simulink model "DiscreteDiffSwerveModuleSimulation"  (R2022a)
settings: Solver=VariableStepAuto  StartTime=0.0  StopTime=2.0  RelTol=1e-3
values from neighbouring files (symbols this model uses):
  Kff = pinv(sysd.B)    [DiffSwerveChassis.m]    (also in GetDiffSwerveModule.m; RunDiffSwerveSimulation.m)
  lqr_K = lqr(sysd, Q, R)    [DiffSwerveChassis.m]    (also in GetDiffSwerveModule.m; RunDiffSwerveSimulation.m)
  sysd = c2d(sysc, Ts)    [DiffSwerveChassis.m]    (also in GetDiffSwerveModule.m; RunDiffSwerveSimulation.m)
  Ts = 0.005    [DiffSwerveChassis.m]    (also in GetDiffSwerveModule.m; RunDiffSwerveSimulation.m)
settings Model: Creator=benjaminwarwick  LastModifiedBy=woz4t

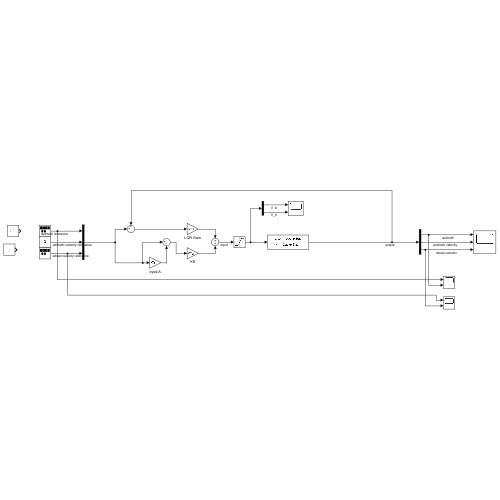
[thumbnail: Simulink's stored preview of the top-level diagram]
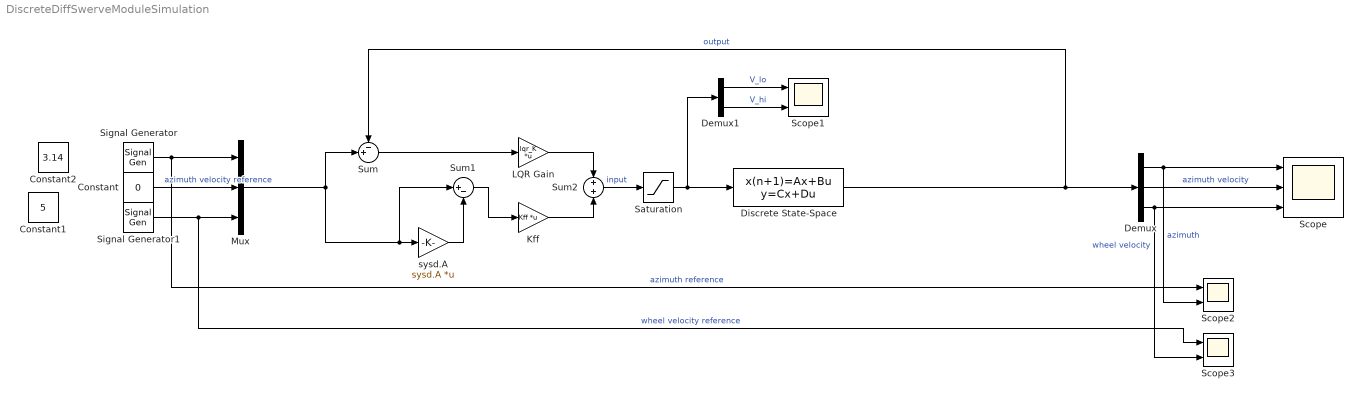
== system DiscreteDiffSwerveModuleSimulation ==
  Constant : Constant  Value=0
  Constant1 : Constant  Value=5
  Constant2 : Constant  Value=3.14
  Demux : Demux  Outputs=3
  Demux1 : Demux  Outputs=2
  Discrete State-Space : DiscreteStateSpace  A=sysd.A  B=sysd.B  C=sysd.C  D=sysd.D  SampleTime=Ts
  Kff : Gain  Gain=Kff  Multiplication=Matrix(K*u)
  LQR Gain : Gain  Gain=lqr_K  Multiplication=Matrix(K*u)
  Mux : Mux  Inputs=3
  Saturation : Saturate  UpperLimit=12  LowerLimit=-12
  Scope : Scope  NumInputPorts=3
  Scope1 : Scope  NumInputPorts=2
  Scope2 : Scope  NumInputPorts=2
  Scope3 : Scope  NumInputPorts=2
  Signal Generator : SignalGenerator  WaveForm=square  Amplitude=3.14  Frequency=20  Units=rad/sec
  Signal Generator1 : SignalGenerator  WaveForm=square  Amplitude=5  Frequency=20  Units=rad/sec
  Sum : Sum  Inputs=-+|
  Sum1 : Sum  Inputs=|+-
  Sum2 : Sum
  sysd.A : Gain  Gain=sysd.A  Multiplication=Matrix(K*u)
  wires:
  Discrete State-Space/1 -> Sum/1, Demux/1  "output"
  Demux/1 -> Scope2/2, Scope/1  "azimuth"
  Demux/2 -> Scope/2  "azimuth velocity"
  Demux/3 -> Scope3/2, Scope/3  "wheel velocity"
  Constant/1 -> Mux/2  "azimuth velocity reference"
  Signal Generator1/1 -> Scope3/1, Mux/3  "wheel velocity reference"
  Mux/1 -> Sum/2, Sum1/1, sysd.A/1
  Sum2/1 -> Saturation/1  "input"
  Demux1/1 -> Scope1/1  "V_lo"
  Demux1/2 -> Scope1/2  "V_hi"
  Signal Generator/1 -> Scope2/1, Mux/1  "azimuth reference"
  Saturation/1 -> Discrete State-Space/1, Demux1/1
  Kff/1 -> Sum2/2
  LQR Gain/1 -> Sum2/1
  sysd.A/1 -> Sum1/2
  Sum1/1 -> Kff/1
  Sum/1 -> LQR Gain/1
